simulink model "GantryRobot"  (R2024a)
settings: Solver=VariableStepAuto  StartTime=0.0  StopTime=10.0  RelTol=1e-3
libraries: simulink x4, sm_lib x3, nesl_utility x1
settings Model: Creator=abirdas  LastModifiedBy=abirdas

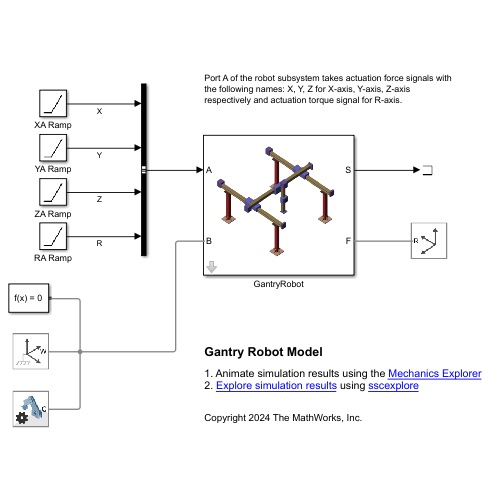
[thumbnail: Simulink's stored preview of the top-level diagram]
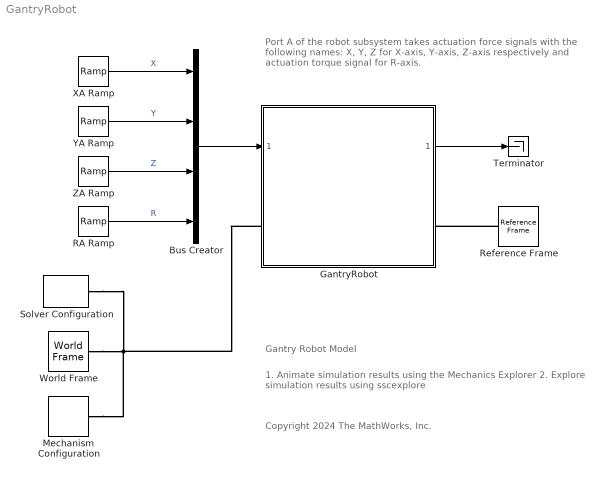
== system GantryRobot ==
  note: Port A of the robot subsystem takes actuation force signals with the following names: X, Y, Z for X-axis, Y-axis, Z-axis respectively and actuation torque signal for R-axis.
  note: 1. Animate simulation results using the Mechanics Explorer
      | 2. Explore simulation results using sscexplore
  note: Copyright 2024 The MathWorks, Inc.
  note: Gantry Robot Model
  Bus Creator : BusCreator  Inputs=4
  GantryRobot : Subsystem  ReferencedSubsystem=GantryRobotSubsystem  DOF=3DOF  configAxis=XYZ  heightColumn=1.2  widthColumn=0.15  positionColumn1=[-1.5,-1.5,0]  positionColumn2=[1.5,-1.5,0]  positionColumn3=[-1.5,1.5,0]  positionColumn4=[1.5,1.5,0]  systemGuideX=Rail-block  strokeXMax=3  widthGuideX=0.15  diaScrewX=0.05  widthXMount=0.3  typeInertiaGuideX=Calculate from Geometry  densityGuideX=2700  massGuideX=0  COMGuideX=0  MOIGuideX=0  POIGuideX=0  typeInertiaCarriageX=Calculate from Geometry  densityCarriageX=2700  massCarriageX=0  COMCarriageX=0  MOICarriageX=0  POICarriageX=0  colorGuideX=[0.7 0.6 0.4]  colorCarriageX=[0.5 0.5 0.9]  systemGuideY=Rail-block  strokeYMax=3  widthGuideY=0.15  diaScrewY=0.05  widthYMount=0.15  typeInertiaGuideY=Calculate from Geometry  densityGuideY=2700  massGuideY=0  COMGuideY=0  MOIGuideY=0  POIGuideY=0  typeInertiaCarriageY=Calculate from Geometry  densityCarriageY=2700  massCarriageY=0  COMCarriageY=0  MOICarriageY=0  POICarriageY=0  colorGuideY=[0.7 0.6 0.4]  colorCarriageY=[0.5 0.5 0.9]  systemGuideZ=Rail-block  strokeZMax=0.9  widthGuideZ=0.15  diaScrewZ=0.05  shiftZAxisDown=0.45  widthZMount=0.15  typeInertiaGuideZ=Calculate from Geometry  densityGuideZ=2700  massGuideZ=0  COMGuideZ=0  MOIGuideZ=0  POIGuideZ=0  typeInertiaCarriageZ=Calculate from Geometry  densityCarriageZ=2700  massCarriageZ=0  COMCarriageZ=0  MOICarriageZ=0  POICarriageZ=0  colorGuideZ=[0.7 0.6 0.4]  colorCarriageZ=[0.5 0.5 0.9]
  Mechanism Configuration : sm_lib/Utilities/Mechanism Configuration  UniformGravity=Constant  GravityVector=[0 0 -9.80665]  GravityVectorUnits=m/s^2  LinearizationDelta=0.001  JointModeTransitionNonlinearIterations=2
  RA Ramp : simulink/Sources/Ramp  slope=0.1  start=0  InitialOutput=0
  Reference Frame : sm_lib/Frames and Transforms/Reference Frame
  Solver Configuration : nesl_utility/Solver Configuration  PhysicalDomain=network_engine_domain  SubClassName=solver  LeftPortType=input  RightPortType=generic  Tones=[]  Harmonics=[]  SimulateNoise=off  Profile=off  UseLocalSampling=off  EnableSwitchedLinearOptims=on  FrequencyDomain=off  UseCCode=off  RelTol=0.001  AbsTol=0.001  MinStep=1e-09  ToWorkspace=off  RevertToSquareIcSolve=off  NumHomotopyIterations=100  PhasorMode=off  PhasorModeNumHarmonics=1  ConsistencySolver=NEWTON_XTOL_AFTER_FTOL  IndexReductionMethod=DerivativeReplacement  DoDC=off  ResidualTolerance=1e-09  ConsistencyTolSource=GLOBAL  ConsistencyAbsTol=0.001  ConsistencyRelTol=0.001  ConsistencyTolFactor=0.001  UseLocalSolver=off  LocalSolverChoice=NE_BACKWARD_EULER_ADVANCER  ResolveIndetEquations=on  FunctionEvalNumThread=1  LocalSolverSampleTime=0.001  DoFixedCost=off  MaxNonlinIter=3  MaxModeIter=2  ComputeImpulses=off  ImpulseIterations=2  LinearAlgebra=auto  LinearAlgebraNumThread=0  EquationFormulation=NE_TIME_EF  DelaysMemoryBudget=1024  AutomaticFiltering=on  FilteringTimeConstant=0.001  PartitionStorageMethod=AS_NEEDED  PartitionMemoryBudget=1024  PartitionMethod=ROBUST  MultibodyUseLocalSolver=off  MultibodyLocalSolverChoice=ODE1  MultibodyLocalSolverSampleTime=0.001
  Terminator : Terminator
  World Frame : sm_lib/Frames and Transforms/World Frame
  XA Ramp : simulink/Sources/Ramp  slope=0.1  start=0  InitialOutput=0
  YA Ramp : simulink/Sources/Ramp  slope=0.1  start=0  InitialOutput=0
  ZA Ramp : simulink/Sources/Ramp  slope=0.1  start=0  InitialOutput=0
  wires:
  GantryRobot/1 -> Terminator/1
  YA Ramp/1 -> Bus Creator/2  "Y"
  RA Ramp/1 -> Bus Creator/4  "R"
  XA Ramp/1 -> Bus Creator/1  "X"
  ZA Ramp/1 -> Bus Creator/3  "Z"
  Bus Creator/1 -> GantryRobot/1
  connections:
  World Frame/RConn1 -- GantryRobot/LConn1 -- Mechanism Configuration/RConn1 -- Solver Configuration/RConn1
  Reference Frame/RConn1 -- GantryRobot/RConn1
